simulink model "SS_angulo_pos_planta_simulink"  (R2023b)
settings: Solver=VariableStepAuto  StartTime=0.0  StopTime=15  RelTol=1e-6
undefined symbols (not defined in the file or in its folder): A, B, C, K_acker, ki_acker
settings Model: Creator=natih  LastModifiedBy=jmarin

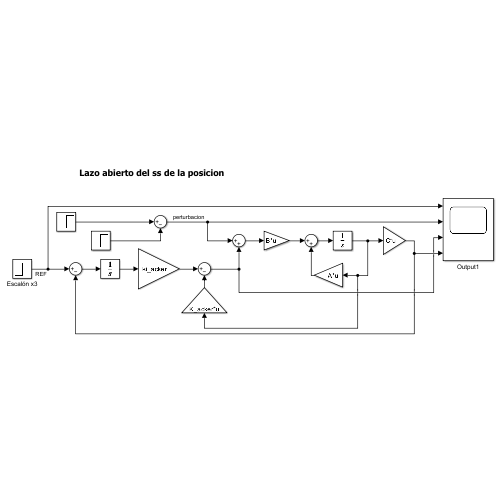
[thumbnail: Simulink's stored preview of the top-level diagram]
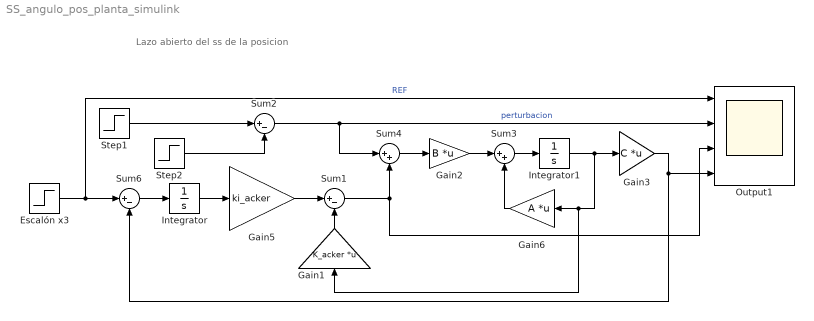
== system SS_angulo_pos_planta_simulink ==
  note: Lazo abierto del ss de la posicion
  Escalón x3 : Step  Time=0.5  After=0.6  SampleTime=0
  Gain1 : Gain  Gain=K_acker  Multiplication=Matrix(K*u)
  Gain2 : Gain  Gain=B  Multiplication=Matrix(K*u)
  Gain3 : Gain  Gain=C  Multiplication=Matrix(K*u)
  Gain5 : Gain  Gain=ki_acker
  Gain6 : Gain  Gain=A  Multiplication=Matrix(K*u)
  Integrator : Integrator
  Integrator1 : Integrator
  Output1 : Scope  NumInputPorts=4
  Step1 : Step  Time=6  After=0.3  SampleTime=0
  Step2 : Step  Time=11  After=0.3  SampleTime=0
  Sum1 : Sum  Inputs=|+-
  Sum2 : Sum  Inputs=|+-
  Sum3 : Sum  Inputs=|++
  Sum4 : Sum  Inputs=|++
  Sum6 : Sum  Inputs=|+-
  wires:
  Step1/1 -> Sum2/1
  Escalón x3/1 -> Output1/1, Sum6/1  "REF"
  Step2/1 -> Sum2/2
  Sum6/1 -> Integrator/1
  Integrator/1 -> Gain5/1
  Gain5/1 -> Sum1/1
  Gain2/1 -> Sum3/1
  Sum3/1 -> Integrator1/1
  Integrator1/1 -> Gain6/1, Gain1/1, Gain3/1
  Gain3/1 -> Sum6/2, Output1/4
  Gain1/1 -> Sum1/2
  Gain6/1 -> Sum3/2
  Sum2/1 -> Sum4/1, Output1/2  "perturbacion"
  Sum1/1 -> Sum4/2, Output1/3
  Sum4/1 -> Gain2/1
